simulink model "Coil5"  (Simulink 7.3)
settings: Solver=ode23tb  StartTime=0.0  StopTime=7/60  RelTol=1e-3
libraries: powerlib x163
settings Model: Creator=DIVYA  LastModifiedBy=intel

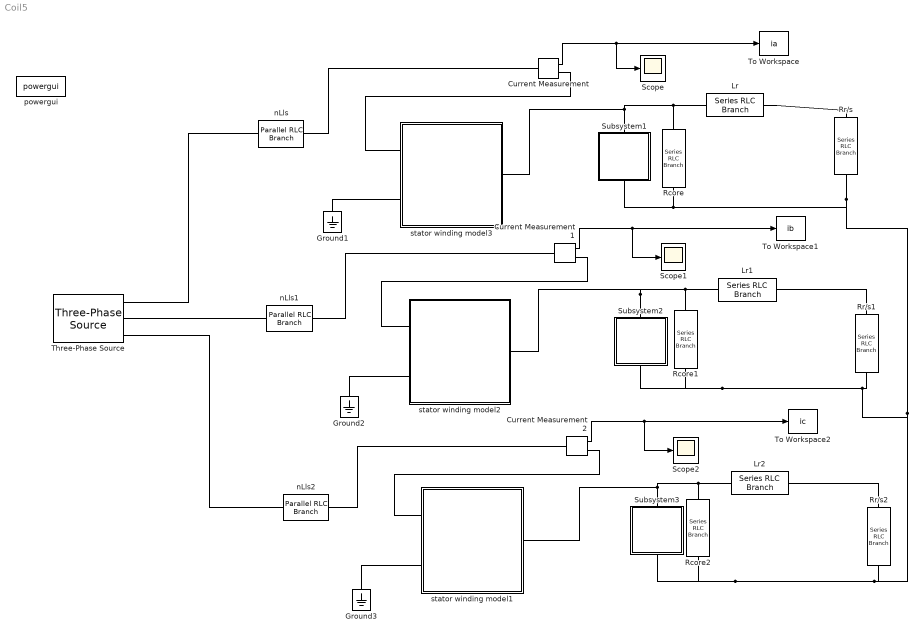
== system Coil5 ==
  Current Measurement : powerlib/Measurements/Current Measurement  DialogController=POWERSYS.PowerSysDialog  SystemSampleTime=-1  PhasorSimulation=off  OutputType=Complex  PSBequivalent=0
  Current Measurement1 : powerlib/Measurements/Current Measurement  DialogController=POWERSYS.PowerSysDialog  SystemSampleTime=-1  PhasorSimulation=off  OutputType=Complex  PSBequivalent=0
  Current Measurement2 : powerlib/Measurements/Current Measurement  DialogController=POWERSYS.PowerSysDialog  SystemSampleTime=-1  PhasorSimulation=off  OutputType=Complex  PSBequivalent=0
  Ground1 : powerlib/Elements/Ground  DialogController=POWERSYS.PowerSysDialog  PhysicalDomain=powersysdomain  SubClassName=unknown  LeftPortType=p1  RightPortType=p1  LConnTagsString=a
  Ground2 : powerlib/Elements/Ground  DialogController=POWERSYS.PowerSysDialog  PhysicalDomain=powersysdomain  SubClassName=unknown  LeftPortType=p1  RightPortType=p1  LConnTagsString=a
  Ground3 : powerlib/Elements/Ground  DialogController=POWERSYS.PowerSysDialog  PhysicalDomain=powersysdomain  SubClassName=unknown  LeftPortType=p1  RightPortType=p1  LConnTagsString=a
  Lr : powerlib/Elements/Series RLC Branch  DialogController=POWERSYS.PowerSysDialog  PhysicalDomain=powersysdomain  SubClassName=unknown  LeftPortType=p1  RightPortType=p1  LConnTagsString=__new0  RConnTagsString=__new0  BranchType=L  Resistance=1.0  Inductance=15.04e-3  SetiL0=off  InitialCurrent=0  Capacitance=1.0  Setx0=off  InitialVoltage=0  Measurements=None
  Lr1 : powerlib/Elements/Series RLC Branch  DialogController=POWERSYS.PowerSysDialog  PhysicalDomain=powersysdomain  SubClassName=unknown  LeftPortType=p1  RightPortType=p1  LConnTagsString=__new0  RConnTagsString=__new0  BranchType=L  Resistance=1.0  Inductance=15.04e-3  SetiL0=off  InitialCurrent=0  Capacitance=1.0  Setx0=off  InitialVoltage=0  Measurements=None
  Lr2 : powerlib/Elements/Series RLC Branch  DialogController=POWERSYS.PowerSysDialog  PhysicalDomain=powersysdomain  SubClassName=unknown  LeftPortType=p1  RightPortType=p1  LConnTagsString=__new0  RConnTagsString=__new0  BranchType=L  Resistance=1.0  Inductance=15.04e-3  SetiL0=off  InitialCurrent=0  Capacitance=1.0  Setx0=off  InitialVoltage=0  Measurements=None
  Rcore : powerlib/Elements/Series RLC Branch  DialogController=POWERSYS.PowerSysDialog  PhysicalDomain=powersysdomain  SubClassName=unknown  LeftPortType=p1  RightPortType=p1  LConnTagsString=__new0  RConnTagsString=__new0  BranchType=R  Resistance=2568  Inductance=1.0  SetiL0=off  InitialCurrent=0  Capacitance=1.0  Setx0=off  InitialVoltage=0  Measurements=None
  Rcore1 : powerlib/Elements/Series RLC Branch  DialogController=POWERSYS.PowerSysDialog  PhysicalDomain=powersysdomain  SubClassName=unknown  LeftPortType=p1  RightPortType=p1  LConnTagsString=__new0  RConnTagsString=__new0  BranchType=R  Resistance=2568  Inductance=1.0  SetiL0=off  InitialCurrent=0  Capacitance=1.0  Setx0=off  InitialVoltage=0  Measurements=None
  Rcore2 : powerlib/Elements/Series RLC Branch  DialogController=POWERSYS.PowerSysDialog  PhysicalDomain=powersysdomain  SubClassName=unknown  LeftPortType=p1  RightPortType=p1  LConnTagsString=__new0  RConnTagsString=__new0  BranchType=R  Resistance=2568  Inductance=1.0  SetiL0=off  InitialCurrent=0  Capacitance=1.0  Setx0=off  InitialVoltage=0  Measurements=None
  Rr/s : powerlib/Elements/Series RLC Branch  DialogController=POWERSYS.PowerSysDialog  PhysicalDomain=powersysdomain  SubClassName=unknown  LeftPortType=p1  RightPortType=p1  LConnTagsString=__new0  RConnTagsString=__new0  BranchType=R  Resistance=1.28/0.027  Inductance=1.0  SetiL0=off  InitialCurrent=0  Capacitance=1.0  Setx0=off  InitialVoltage=0  Measurements=None
  Rr/s1 : powerlib/Elements/Series RLC Branch  DialogController=POWERSYS.PowerSysDialog  PhysicalDomain=powersysdomain  SubClassName=unknown  LeftPortType=p1  RightPortType=p1  LConnTagsString=__new0  RConnTagsString=__new0  BranchType=R  Resistance=1.28/0.027  Inductance=1.0  SetiL0=off  InitialCurrent=0  Capacitance=1.0  Setx0=off  InitialVoltage=0  Measurements=None
  Rr/s2 : powerlib/Elements/Series RLC Branch  DialogController=POWERSYS.PowerSysDialog  PhysicalDomain=powersysdomain  SubClassName=unknown  LeftPortType=p1  RightPortType=p1  LConnTagsString=__new0  RConnTagsString=__new0  BranchType=R  Resistance=1.28/0.027  Inductance=1.0  SetiL0=off  InitialCurrent=0  Capacitance=1.0  Setx0=off  InitialVoltage=0  Measurements=None
  Scope : Scope
      settings: YMin=-8  YMax=6  SaveName=ScopeData18
  Scope1 : Scope
      settings: SaveName=ScopeData6
  Scope2 : Scope
      settings: SaveName=ScopeData7
  Subsystem1 : Subsystem
  Subsystem2 : Subsystem
  Subsystem3 : Subsystem
  Three-Phase Source : powerlib/Electrical Sources/Three-Phase Source  DialogController=POWERSYS.PowerSysDialog  SystemSampleTime=-1  Voltage=460  PhaseAngle=0  Frequency=60  InternalConnection=Yg  SpecifyImpedance=on  Resistance=0.8929  Inductance=16.58e-3  ShortCircuitLevel=100e6  BaseVoltage=25e3  XRratio=7
  To Workspace : ToWorkspace  VariableName=ia  SampleTime=1/(60*128)  SaveFormat=Array
  To Workspace1 : ToWorkspace  VariableName=ib  SampleTime=1/(60*128)  SaveFormat=Array
  To Workspace2 : ToWorkspace  VariableName=ic  SampleTime=1/(60*128)  SaveFormat=Array
  nLls : powerlib/Elements/Parallel RLC Branch  DialogController=POWERSYS.PowerSysDialog  PhysicalDomain=powersysdomain  SubClassName=unknown  LeftPortType=p1  RightPortType=p1  LConnTagsString=a  RConnTagsString=__new0  BranchType=L  Resistance=1.0  Inductance=4.926e-6  SetiL0=off  InitialCurrent=0  Capacitance=1.0  Setx0=off  InitialVoltage=0  Measurements=None
  nLls1 : powerlib/Elements/Parallel RLC Branch  DialogController=POWERSYS.PowerSysDialog  PhysicalDomain=powersysdomain  SubClassName=unknown  LeftPortType=p1  RightPortType=p1  LConnTagsString=a  RConnTagsString=__new0  BranchType=L  Resistance=1.0  Inductance=4.926e-6  SetiL0=off  InitialCurrent=0  Capacitance=1.0  Setx0=off  InitialVoltage=0  Measurements=None
  nLls2 : powerlib/Elements/Parallel RLC Branch  DialogController=POWERSYS.PowerSysDialog  PhysicalDomain=powersysdomain  SubClassName=unknown  LeftPortType=p1  RightPortType=p1  LConnTagsString=a  RConnTagsString=__new0  BranchType=L  Resistance=1.0  Inductance=4.926e-6  SetiL0=off  InitialCurrent=0  Capacitance=1.0  Setx0=off  InitialVoltage=0  Measurements=None
  powergui : powerlib/powergui  SystemSampleTime=-1  SimulationMode=Continuous  SampleTime=50e-6  frequency=60  SPID=off  DisableSnubberDevices=off  DisableRonSwitches=off  DisableVfSwitches=off  SwTol=0  Interpol=off  frequencyindice=60  echomessages=off  HookPort=off  DisplayEquations=off  FunctionMessages=off  EnableUseOfTLC=off  x0status=blocks  RestoreLinks=warning  Frange=[0:2:500]  Ylog=off  Xlog=on  ShowGrid=off  save=off  variable=ZData  structure=ScopeData18  ZoomFFT=off  StartTime=0.00  cycles=2  DisplayStyle=1  fundamental=60  FreqAxis=off  MaxFrequency=200  frequencyindicesteady=1  RmsSteady=1  display=off  Ts=0  methode=off
  stator winding model1 : Subsystem
  stator winding model2 : Subsystem
  stator winding model3 : Subsystem
  wires:
  Current Measurement/1 -> To Workspace/1, Scope/1
  Current Measurement1/1 -> To Workspace1/1, Scope1/1
  Current Measurement2/1 -> To Workspace2/1, Scope2/1
  connections:
  Lr/LConn1 -- Rr/s/LConn1
  Current Measurement/LConn1 -- nLls/RConn1
  Current Measurement/RConn1 -- stator winding model3/LConn1
  Three-Phase Source/RConn1 -- nLls/LConn1
  stator winding model3/RConn1 -- Subsystem1/LConn1 -- Lr/RConn1 -- Rcore/LConn1
  stator winding model2/RConn1 -- Subsystem2/LConn1 -- Rcore1/LConn1 -- Lr1/RConn1
  Lr1/LConn1 -- Rr/s1/LConn1
  Current Measurement1/LConn1 -- nLls1/RConn1
  Current Measurement1/RConn1 -- stator winding model2/LConn1
  Ground2/LConn1 -- stator winding model2/LConn2
  Rr/s/RConn1 -- Subsystem2/RConn1 -- Rcore1/RConn1 -- Rr/s1/RConn1 -- Rr/s2/RConn1 -- Rcore2/RConn1 -- Subsystem3/RConn1 -- Subsystem1/RConn1 -- Rcore/RConn1
  stator winding model1/RConn1 -- Subsystem3/LConn1 -- Rcore2/LConn1 -- Lr2/RConn1
  Lr2/LConn1 -- Rr/s2/LConn1
  Current Measurement2/LConn1 -- nLls2/RConn1
  Current Measurement2/RConn1 -- stator winding model1/LConn1
  Ground3/LConn1 -- stator winding model1/LConn2
  Three-Phase Source/RConn2 -- nLls1/LConn1
  Three-Phase Source/RConn3 -- nLls2/LConn1
  Ground1/LConn1 -- stator winding model3/LConn2

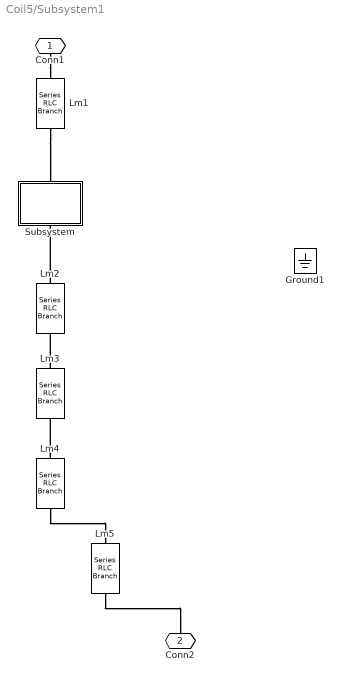
== system Coil5/Subsystem1 ==
  Ground1 : powerlib/Elements/Ground  DialogController=POWERSYS.PowerSysDialog  PhysicalDomain=powersysdomain  SubClassName=unknown  LeftPortType=p1  RightPortType=p1  LConnTagsString=a
  Lm{1..5} (5 alike) : powerlib/Elements/Series RLC Branch  DialogController=POWERSYS.PowerSysDialog  PhysicalDomain=powersysdomain  SubClassName=unknown  LeftPortType=p1  RightPortType=p1  LConnTagsString=__new0  RConnTagsString=__new0  BranchType=L  Resistance=1.0  Inductance=319e-3/6  SetiL0=off  InitialCurrent=0  Capacitance=1.0  Setx0=off  InitialVoltage=0  Measurements=None
  Subsystem : Subsystem
  Conn1 : PMIOPort  Port=1  Side=Left
  Conn2 : PMIOPort  Port=2  Side=Right
  connections:
  Conn1/RConn1 -- Lm1/LConn1
  Lm4/LConn1 -- Lm3/RConn1
  Lm3/LConn1 -- Lm2/RConn1
  Lm2/LConn1 -- Subsystem/RConn1
  Lm1/RConn1 -- Subsystem/LConn1
  Lm4/RConn1 -- Lm5/LConn1
  Lm5/RConn1 -- Conn2/RConn1

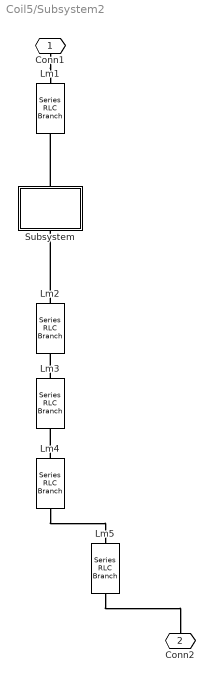
== system Coil5/Subsystem2 ==
  Lm{1..5} (5 alike) : powerlib/Elements/Series RLC Branch  DialogController=POWERSYS.PowerSysDialog  PhysicalDomain=powersysdomain  SubClassName=unknown  LeftPortType=p1  RightPortType=p1  LConnTagsString=__new0  RConnTagsString=__new0  BranchType=L  Resistance=1.0  Inductance=319e-3/6  SetiL0=off  InitialCurrent=0  Capacitance=1.0  Setx0=off  InitialVoltage=0  Measurements=None
  Subsystem : Subsystem
  Conn1 : PMIOPort  Port=1  Side=Left
  Conn2 : PMIOPort  Port=2  Side=Right
  connections:
  Conn1/RConn1 -- Lm1/LConn1
  Lm4/LConn1 -- Lm3/RConn1
  Lm3/LConn1 -- Lm2/RConn1
  Lm2/LConn1 -- Subsystem/RConn1
  Subsystem/LConn1 -- Lm1/RConn1
  Lm4/RConn1 -- Lm5/LConn1
  Lm5/RConn1 -- Conn2/RConn1

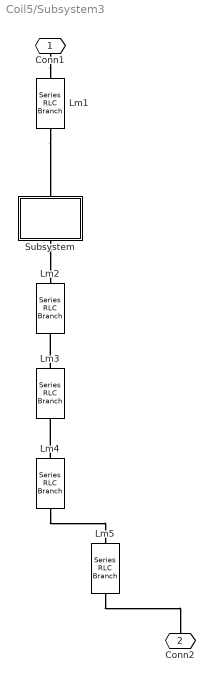
== system Coil5/Subsystem3 ==
  Lm{1..5} (5 alike) : powerlib/Elements/Series RLC Branch  DialogController=POWERSYS.PowerSysDialog  PhysicalDomain=powersysdomain  SubClassName=unknown  LeftPortType=p1  RightPortType=p1  LConnTagsString=__new0  RConnTagsString=__new0  BranchType=L  Resistance=1.0  Inductance=319e-3/6  SetiL0=off  InitialCurrent=0  Capacitance=1.0  Setx0=off  InitialVoltage=0  Measurements=None
  Subsystem : Subsystem
  Conn1 : PMIOPort  Port=1  Side=Left
  Conn2 : PMIOPort  Port=2  Side=Right
  connections:
  Conn1/RConn1 -- Lm1/LConn1
  Lm4/LConn1 -- Lm3/RConn1
  Lm3/LConn1 -- Lm2/RConn1
  Subsystem/RConn1 -- Lm2/LConn1
  Lm1/RConn1 -- Subsystem/LConn1
  Lm4/RConn1 -- Lm5/LConn1
  Lm5/RConn1 -- Conn2/RConn1

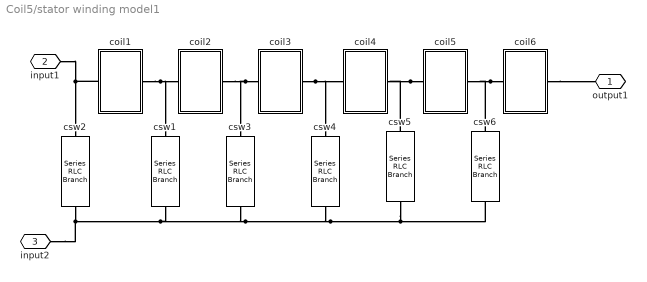
== system Coil5/stator winding model1 ==
  coil1 : Subsystem
  coil2 : Subsystem
  coil3 : Subsystem
  coil4 : Subsystem
  coil5 : Subsystem
  coil6 : Subsystem
  csw{1..6} (6 alike) : powerlib/Elements/Series RLC Branch  DialogController=POWERSYS.PowerSysDialog  PhysicalDomain=powersysdomain  SubClassName=unknown  LeftPortType=p1  RightPortType=p1  LConnTagsString=__new0  RConnTagsString=__new0  BranchType=RC  Resistance=(4*10)/(192*6)  Inductance=1.0  SetiL0=off  InitialCurrent=0  Capacitance=0.213e-9/6  Setx0=off  InitialVoltage=0  Measurements=None
  output1 : PMIOPort  Port=1  Side=Left
  input1 : PMIOPort  Port=2  Side=Right
  input2 : PMIOPort  Port=3  Side=Left
  connections:
  coil1/RConn1 -- coil2/LConn1 -- csw1/LConn1
  coil3/LConn1 -- coil2/RConn1 -- csw3/LConn1
  coil3/RConn1 -- coil4/LConn1 -- csw4/LConn1
  coil5/LConn1 -- csw5/LConn1 -- coil4/RConn1
  coil6/LConn1 -- csw6/LConn1 -- coil5/RConn1
  input2/RConn1 -- csw6/RConn1 -- csw5/RConn1 -- csw4/RConn1 -- csw3/RConn1 -- csw1/RConn1 -- csw2/RConn1
  coil6/RConn1 -- output1/RConn1
  coil1/LConn1 -- csw2/LConn1 -- input1/RConn1

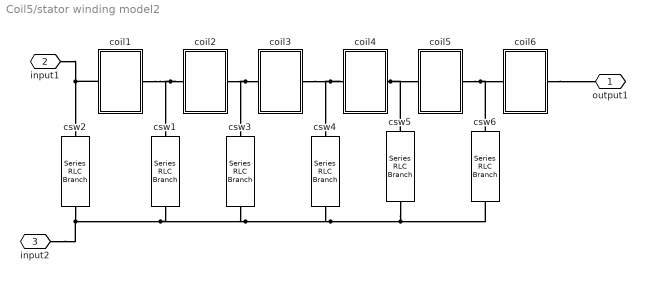
== system Coil5/stator winding model2 ==
  coil1 : Subsystem
  coil2 : Subsystem
  coil3 : Subsystem
  coil4 : Subsystem
  coil5 : Subsystem
  coil6 : Subsystem
  csw{1..6} (6 alike) : powerlib/Elements/Series RLC Branch  DialogController=POWERSYS.PowerSysDialog  PhysicalDomain=powersysdomain  SubClassName=unknown  LeftPortType=p1  RightPortType=p1  LConnTagsString=__new0  RConnTagsString=__new0  BranchType=RC  Resistance=(4*10)/(192*6)  Inductance=1.0  SetiL0=off  InitialCurrent=0  Capacitance=0.213e-9/6  Setx0=off  InitialVoltage=0  Measurements=None
  output1 : PMIOPort  Port=1  Side=Left
  input1 : PMIOPort  Port=2  Side=Right
  input2 : PMIOPort  Port=3  Side=Left
  connections:
  coil2/LConn1 -- csw1/LConn1 -- coil1/RConn1
  coil3/LConn1 -- csw3/LConn1 -- coil2/RConn1
  coil4/LConn1 -- csw4/LConn1 -- coil3/RConn1
  coil4/RConn1 -- csw5/LConn1 -- coil5/LConn1
  coil5/RConn1 -- coil6/LConn1 -- csw6/LConn1
  input2/RConn1 -- csw6/RConn1 -- csw5/RConn1 -- csw4/RConn1 -- csw3/RConn1 -- csw1/RConn1 -- csw2/RConn1
  coil6/RConn1 -- output1/RConn1
  coil1/LConn1 -- csw2/LConn1 -- input1/RConn1

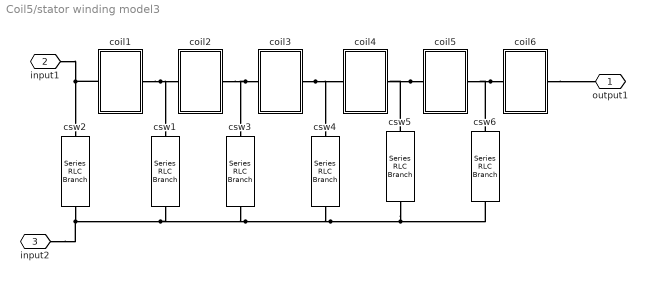
== system Coil5/stator winding model3 ==
  coil1 : Subsystem
  coil2 : Subsystem
  coil3 : Subsystem
  coil4 : Subsystem
  coil5 : Subsystem
  coil6 : Subsystem
  csw{1..6} (6 alike) : powerlib/Elements/Series RLC Branch  DialogController=POWERSYS.PowerSysDialog  PhysicalDomain=powersysdomain  SubClassName=unknown  LeftPortType=p1  RightPortType=p1  LConnTagsString=__new0  RConnTagsString=__new0  BranchType=RC  Resistance=(4*10)/(192*6)  Inductance=1.0  SetiL0=off  InitialCurrent=0  Capacitance=0.213e-9/6  Setx0=off  InitialVoltage=0  Measurements=None
  output1 : PMIOPort  Port=1  Side=Left
  input1 : PMIOPort  Port=2  Side=Right
  input2 : PMIOPort  Port=3  Side=Left
  connections:
  coil1/RConn1 -- coil2/LConn1 -- csw1/LConn1
  coil3/LConn1 -- coil2/RConn1 -- csw3/LConn1
  coil3/RConn1 -- coil4/LConn1 -- csw4/LConn1
  coil5/LConn1 -- csw5/LConn1 -- coil4/RConn1
  coil6/LConn1 -- csw6/LConn1 -- coil5/RConn1
  input2/RConn1 -- csw6/RConn1 -- csw5/RConn1 -- csw4/RConn1 -- csw3/RConn1 -- csw1/RConn1 -- csw2/RConn1
  coil6/RConn1 -- output1/RConn1
  coil1/LConn1 -- csw2/LConn1 -- input1/RConn1

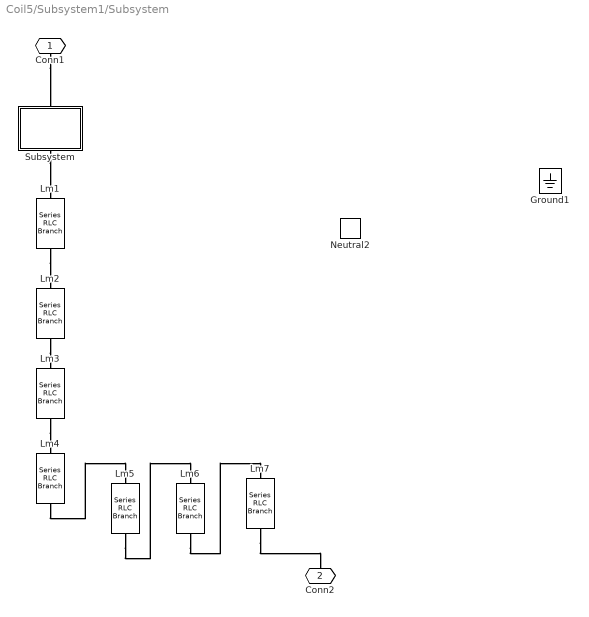
== system Coil5/Subsystem1/Subsystem ==
  Ground1 : powerlib/Elements/Ground  DialogController=POWERSYS.PowerSysDialog  PhysicalDomain=powersysdomain  SubClassName=unknown  LeftPortType=p1  RightPortType=p1  LConnTagsString=a
  Lm{1..7} (7 alike) : powerlib/Elements/Series RLC Branch  DialogController=POWERSYS.PowerSysDialog  PhysicalDomain=powersysdomain  SubClassName=unknown  LeftPortType=p1  RightPortType=p1  LConnTagsString=__new0  RConnTagsString=__new0  BranchType=L  Resistance=1.0  Inductance=319e-3/(8*6)  SetiL0=off  InitialCurrent=0  Capacitance=1.0  Setx0=off  InitialVoltage=0  Measurements=None
  Neutral2 : powerlib/Elements/Neutral  DialogController=POWERSYS.PowerSysDialog  PhysicalDomain=powersysdomain  SubClassName=unknown  LeftPortType=p1  RightPortType=p1  LConnTagsString=a  NodeNumber=20
  Subsystem : Subsystem
  Conn1 : PMIOPort  Port=1  Side=Left
  Conn2 : PMIOPort  Port=2  Side=Right
  connections:
  Lm1/RConn1 -- Lm2/LConn1
  Lm2/RConn1 -- Lm3/LConn1
  Lm3/RConn1 -- Lm4/LConn1
  Lm4/RConn1 -- Lm5/RConn1
  Lm5/LConn1 -- Lm6/RConn1
  Lm6/LConn1 -- Lm7/LConn1
  Lm7/RConn1 -- Conn2/RConn1
  Conn1/RConn1 -- Subsystem/LConn1
  Subsystem/RConn1 -- Lm1/LConn1

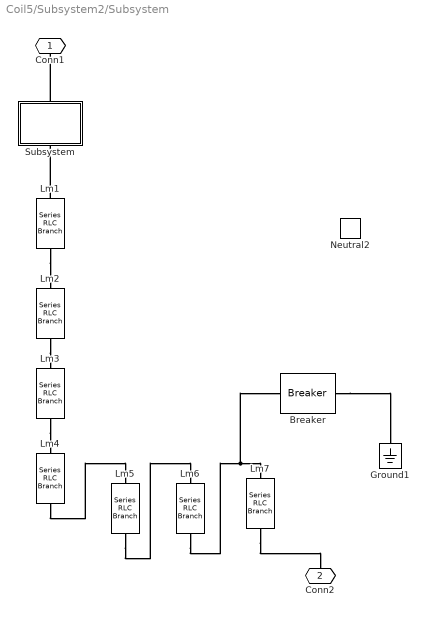
== system Coil5/Subsystem2/Subsystem ==
  Breaker : powerlib/Elements/Breaker  DialogController=POWERSYS.PowerSysDialog  SystemSampleTime=-1  BreakerResistance=0.01  InitialState=0  SnubberResistance=1e6  SnubberCapacitance=inf  SwitchingTimes="[ 3/60  20/60 ]"  External=off  Measurements=None  MoreParameters=off  NoBreakLoop=off
  Ground1 : powerlib/Elements/Ground  DialogController=POWERSYS.PowerSysDialog  PhysicalDomain=powersysdomain  SubClassName=unknown  LeftPortType=p1  RightPortType=p1  LConnTagsString=a
  Lm{1..7} (7 alike) : powerlib/Elements/Series RLC Branch  DialogController=POWERSYS.PowerSysDialog  PhysicalDomain=powersysdomain  SubClassName=unknown  LeftPortType=p1  RightPortType=p1  LConnTagsString=__new0  RConnTagsString=__new0  BranchType=L  Resistance=1.0  Inductance=319e-3/(8*6)  SetiL0=off  InitialCurrent=0  Capacitance=1.0  Setx0=off  InitialVoltage=0  Measurements=None
  Neutral2 : powerlib/Elements/Neutral  DialogController=POWERSYS.PowerSysDialog  PhysicalDomain=powersysdomain  SubClassName=unknown  LeftPortType=p1  RightPortType=p1  LConnTagsString=a  NodeNumber=20
  Subsystem : Subsystem
  Conn1 : PMIOPort  Port=1  Side=Left
  Conn2 : PMIOPort  Port=2  Side=Right
  connections:
  Lm1/RConn1 -- Lm2/LConn1
  Lm2/RConn1 -- Lm3/LConn1
  Lm3/RConn1 -- Lm4/LConn1
  Lm4/RConn1 -- Lm5/RConn1
  Lm5/LConn1 -- Lm6/RConn1
  Lm6/LConn1 -- Lm7/LConn1 -- Breaker/LConn1
  Lm7/RConn1 -- Conn2/RConn1
  Subsystem/LConn1 -- Conn1/RConn1
  Lm1/LConn1 -- Subsystem/RConn1
  Breaker/RConn1 -- Ground1/LConn1

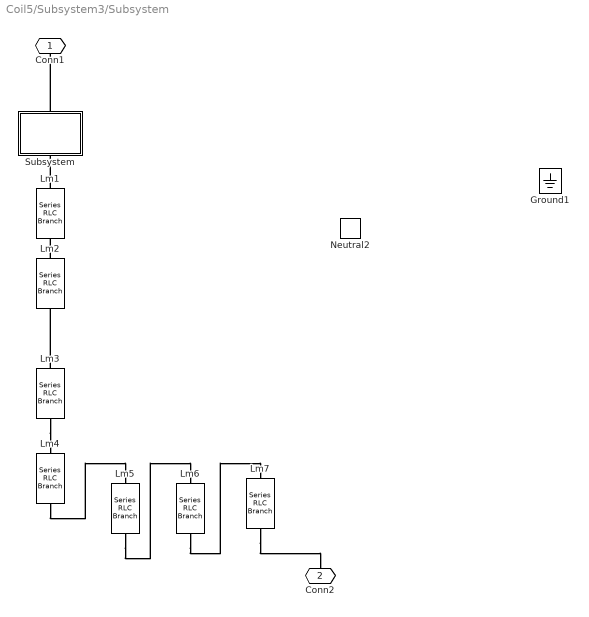
== system Coil5/Subsystem3/Subsystem ==
  Ground1 : powerlib/Elements/Ground  DialogController=POWERSYS.PowerSysDialog  PhysicalDomain=powersysdomain  SubClassName=unknown  LeftPortType=p1  RightPortType=p1  LConnTagsString=a
  Lm{1..7} (7 alike) : powerlib/Elements/Series RLC Branch  DialogController=POWERSYS.PowerSysDialog  PhysicalDomain=powersysdomain  SubClassName=unknown  LeftPortType=p1  RightPortType=p1  LConnTagsString=__new0  RConnTagsString=__new0  BranchType=L  Resistance=1.0  Inductance=319e-3/(8*6)  SetiL0=off  InitialCurrent=0  Capacitance=1.0  Setx0=off  InitialVoltage=0  Measurements=None
  Neutral2 : powerlib/Elements/Neutral  DialogController=POWERSYS.PowerSysDialog  PhysicalDomain=powersysdomain  SubClassName=unknown  LeftPortType=p1  RightPortType=p1  LConnTagsString=a  NodeNumber=20
  Subsystem : Subsystem
  Conn1 : PMIOPort  Port=1  Side=Left
  Conn2 : PMIOPort  Port=2  Side=Right
  connections:
  Lm2/LConn1 -- Lm1/RConn1
  Lm3/LConn1 -- Lm2/RConn1
  Lm3/RConn1 -- Lm4/LConn1
  Lm4/RConn1 -- Lm5/RConn1
  Lm5/LConn1 -- Lm6/RConn1
  Lm6/LConn1 -- Lm7/LConn1
  Lm7/RConn1 -- Conn2/RConn1
  Subsystem/LConn1 -- Conn1/RConn1
  Lm1/LConn1 -- Subsystem/RConn1

== system Coil5/stator winding model1/coil1 ==
  Ground : powerlib/Elements/Ground  DialogController=POWERSYS.PowerSysDialog  PhysicalDomain=powersysdomain  SubClassName=unknown  LeftPortType=p1  RightPortType=p1  LConnTagsString=a
  LC Branch1 : powerlib/Elements/Parallel RLC Branch  DialogController=POWERSYS.PowerSysDialog  PhysicalDomain=powersysdomain  SubClassName=unknown  LeftPortType=p1  RightPortType=p1  LConnTagsString=a  RConnTagsString=__new0  BranchType=RLC  Resistance=11.867e3/6  Inductance=(11.35E-3)/6  SetiL0=off  InitialCurrent=0  Capacitance=0.852e-9*6  Setx0=off  InitialVoltage=0  Measurements=None
  Rs1 : powerlib/Elements/Parallel RLC Branch  DialogController=POWERSYS.PowerSysDialog  PhysicalDomain=powersysdomain  SubClassName=unknown  LeftPortType=p1  RightPortType=p1  LConnTagsString=a  RConnTagsString=__new0  BranchType=R  Resistance=1.41/6  Inductance=1.0  SetiL0=off  InitialCurrent=0  Capacitance=1.0  Setx0=off  InitialVoltage=0  Measurements=None
  Conn1 : PMIOPort  Port=1  Side=Left
  Conn2 : PMIOPort  Port=2  Side=Right
  connections:
  Rs1/LConn1 -- Conn1/RConn1
  LC Branch1/RConn1 -- Conn2/RConn1
  Rs1/RConn1 -- LC Branch1/LConn1

== system Coil5/stator winding model1/coil2 ==
  Ground : powerlib/Elements/Ground  DialogController=POWERSYS.PowerSysDialog  PhysicalDomain=powersysdomain  SubClassName=unknown  LeftPortType=p1  RightPortType=p1  LConnTagsString=a
  LC Branch1 : powerlib/Elements/Parallel RLC Branch  DialogController=POWERSYS.PowerSysDialog  PhysicalDomain=powersysdomain  SubClassName=unknown  LeftPortType=p1  RightPortType=p1  LConnTagsString=a  RConnTagsString=__new0  BranchType=RLC  Resistance=11.867e3/6  Inductance=(11.35E-3)/6  SetiL0=off  InitialCurrent=0  Capacitance=0.852e-9*6  Setx0=off  InitialVoltage=0  Measurements=None
  Rs1 : powerlib/Elements/Parallel RLC Branch  DialogController=POWERSYS.PowerSysDialog  PhysicalDomain=powersysdomain  SubClassName=unknown  LeftPortType=p1  RightPortType=p1  LConnTagsString=a  RConnTagsString=__new0  BranchType=R  Resistance=1.41/6  Inductance=1.0  SetiL0=off  InitialCurrent=0  Capacitance=1.0  Setx0=off  InitialVoltage=0  Measurements=None
  Conn1 : PMIOPort  Port=1  Side=Left
  Conn2 : PMIOPort  Port=2  Side=Right
  connections:
  Rs1/LConn1 -- Conn1/RConn1
  LC Branch1/RConn1 -- Conn2/RConn1
  Rs1/RConn1 -- LC Branch1/LConn1

== system Coil5/stator winding model1/coil3 ==
  Ground : powerlib/Elements/Ground  DialogController=POWERSYS.PowerSysDialog  PhysicalDomain=powersysdomain  SubClassName=unknown  LeftPortType=p1  RightPortType=p1  LConnTagsString=a
  LC Branch1 : powerlib/Elements/Parallel RLC Branch  DialogController=POWERSYS.PowerSysDialog  PhysicalDomain=powersysdomain  SubClassName=unknown  LeftPortType=p1  RightPortType=p1  LConnTagsString=a  RConnTagsString=__new0  BranchType=RLC  Resistance=11.867e3/6  Inductance=(11.35E-3)/6  SetiL0=off  InitialCurrent=0  Capacitance=0.852e-9*6  Setx0=off  InitialVoltage=0  Measurements=None
  Rs1 : powerlib/Elements/Parallel RLC Branch  DialogController=POWERSYS.PowerSysDialog  PhysicalDomain=powersysdomain  SubClassName=unknown  LeftPortType=p1  RightPortType=p1  LConnTagsString=a  RConnTagsString=__new0  BranchType=R  Resistance=1.41/6  Inductance=1.0  SetiL0=off  InitialCurrent=0  Capacitance=1.0  Setx0=off  InitialVoltage=0  Measurements=None
  Conn1 : PMIOPort  Port=1  Side=Left
  Conn2 : PMIOPort  Port=2  Side=Right
  connections:
  Rs1/LConn1 -- Conn1/RConn1
  LC Branch1/RConn1 -- Conn2/RConn1
  Rs1/RConn1 -- LC Branch1/LConn1

== system Coil5/stator winding model1/coil4 ==
  Ground : powerlib/Elements/Ground  DialogController=POWERSYS.PowerSysDialog  PhysicalDomain=powersysdomain  SubClassName=unknown  LeftPortType=p1  RightPortType=p1  LConnTagsString=a
  LC Branch1 : powerlib/Elements/Parallel RLC Branch  DialogController=POWERSYS.PowerSysDialog  PhysicalDomain=powersysdomain  SubClassName=unknown  LeftPortType=p1  RightPortType=p1  LConnTagsString=a  RConnTagsString=__new0  BranchType=RLC  Resistance=11.867e3/6  Inductance=(11.35E-3)/6  SetiL0=off  InitialCurrent=0  Capacitance=0.852e-9*6  Setx0=off  InitialVoltage=0  Measurements=None
  Rs1 : powerlib/Elements/Parallel RLC Branch  DialogController=POWERSYS.PowerSysDialog  PhysicalDomain=powersysdomain  SubClassName=unknown  LeftPortType=p1  RightPortType=p1  LConnTagsString=a  RConnTagsString=__new0  BranchType=R  Resistance=1.41/6  Inductance=1.0  SetiL0=off  InitialCurrent=0  Capacitance=1.0  Setx0=off  InitialVoltage=0  Measurements=None
  Conn1 : PMIOPort  Port=1  Side=Left
  Conn2 : PMIOPort  Port=2  Side=Right
  connections:
  Rs1/LConn1 -- Conn1/RConn1
  LC Branch1/RConn1 -- Conn2/RConn1
  Rs1/RConn1 -- LC Branch1/LConn1

== system Coil5/stator winding model1/coil5 ==
  Ground : powerlib/Elements/Ground  DialogController=POWERSYS.PowerSysDialog  PhysicalDomain=powersysdomain  SubClassName=unknown  LeftPortType=p1  RightPortType=p1  LConnTagsString=a
  LC Branch1 : powerlib/Elements/Parallel RLC Branch  DialogController=POWERSYS.PowerSysDialog  PhysicalDomain=powersysdomain  SubClassName=unknown  LeftPortType=p1  RightPortType=p1  LConnTagsString=a  RConnTagsString=__new0  BranchType=RLC  Resistance=11.867e3/6  Inductance=(11.35E-3)/6  SetiL0=off  InitialCurrent=0  Capacitance=0.852e-9*6  Setx0=off  InitialVoltage=0  Measurements=None
  Rs1 : powerlib/Elements/Parallel RLC Branch  DialogController=POWERSYS.PowerSysDialog  PhysicalDomain=powersysdomain  SubClassName=unknown  LeftPortType=p1  RightPortType=p1  LConnTagsString=a  RConnTagsString=__new0  BranchType=R  Resistance=1.41/6  Inductance=1.0  SetiL0=off  InitialCurrent=0  Capacitance=1.0  Setx0=off  InitialVoltage=0  Measurements=None
  Conn1 : PMIOPort  Port=1  Side=Left
  Conn2 : PMIOPort  Port=2  Side=Right
  connections:
  Rs1/LConn1 -- Conn1/RConn1
  LC Branch1/RConn1 -- Conn2/RConn1
  Rs1/RConn1 -- LC Branch1/LConn1

== system Coil5/stator winding model1/coil6 ==
  Ground : powerlib/Elements/Ground  DialogController=POWERSYS.PowerSysDialog  PhysicalDomain=powersysdomain  SubClassName=unknown  LeftPortType=p1  RightPortType=p1  LConnTagsString=a
  LC Branch1 : powerlib/Elements/Parallel RLC Branch  DialogController=POWERSYS.PowerSysDialog  PhysicalDomain=powersysdomain  SubClassName=unknown  LeftPortType=p1  RightPortType=p1  LConnTagsString=a  RConnTagsString=__new0  BranchType=RLC  Resistance=11.867e3/6  Inductance=(11.35E-3)/6  SetiL0=off  InitialCurrent=0  Capacitance=0.852e-9*6  Setx0=off  InitialVoltage=0  Measurements=None
  Rs1 : powerlib/Elements/Parallel RLC Branch  DialogController=POWERSYS.PowerSysDialog  PhysicalDomain=powersysdomain  SubClassName=unknown  LeftPortType=p1  RightPortType=p1  LConnTagsString=a  RConnTagsString=__new0  BranchType=R  Resistance=1.41/6  Inductance=1.0  SetiL0=off  InitialCurrent=0  Capacitance=1.0  Setx0=off  InitialVoltage=0  Measurements=None
  Conn1 : PMIOPort  Port=1  Side=Left
  Conn2 : PMIOPort  Port=2  Side=Right
  connections:
  Rs1/LConn1 -- Conn1/RConn1
  LC Branch1/RConn1 -- Conn2/RConn1
  Rs1/RConn1 -- LC Branch1/LConn1

== system Coil5/stator winding model2/coil1 ==
  Ground : powerlib/Elements/Ground  DialogController=POWERSYS.PowerSysDialog  PhysicalDomain=powersysdomain  SubClassName=unknown  LeftPortType=p1  RightPortType=p1  LConnTagsString=a
  LC Branch1 : powerlib/Elements/Parallel RLC Branch  DialogController=POWERSYS.PowerSysDialog  PhysicalDomain=powersysdomain  SubClassName=unknown  LeftPortType=p1  RightPortType=p1  LConnTagsString=a  RConnTagsString=__new0  BranchType=RLC  Resistance=11.867e3/6  Inductance=(11.35E-3)/6  SetiL0=off  InitialCurrent=0  Capacitance=0.852e-9*6  Setx0=off  InitialVoltage=0  Measurements=None
  Rs1 : powerlib/Elements/Parallel RLC Branch  DialogController=POWERSYS.PowerSysDialog  PhysicalDomain=powersysdomain  SubClassName=unknown  LeftPortType=p1  RightPortType=p1  LConnTagsString=a  RConnTagsString=__new0  BranchType=R  Resistance=1.41/6  Inductance=1.0  SetiL0=off  InitialCurrent=0  Capacitance=1.0  Setx0=off  InitialVoltage=0  Measurements=None
  Conn1 : PMIOPort  Port=1  Side=Left
  Conn2 : PMIOPort  Port=2  Side=Right
  connections:
  Rs1/LConn1 -- Conn1/RConn1
  LC Branch1/RConn1 -- Conn2/RConn1
  Rs1/RConn1 -- LC Branch1/LConn1

== system Coil5/stator winding model2/coil2 ==
  Ground : powerlib/Elements/Ground  DialogController=POWERSYS.PowerSysDialog  PhysicalDomain=powersysdomain  SubClassName=unknown  LeftPortType=p1  RightPortType=p1  LConnTagsString=a
  LC Branch1 : powerlib/Elements/Parallel RLC Branch  DialogController=POWERSYS.PowerSysDialog  PhysicalDomain=powersysdomain  SubClassName=unknown  LeftPortType=p1  RightPortType=p1  LConnTagsString=a  RConnTagsString=__new0  BranchType=RLC  Resistance=11.867e3/6  Inductance=(11.35E-3)/6  SetiL0=off  InitialCurrent=0  Capacitance=0.852e-9*6  Setx0=off  InitialVoltage=0  Measurements=None
  Rs1 : powerlib/Elements/Parallel RLC Branch  DialogController=POWERSYS.PowerSysDialog  PhysicalDomain=powersysdomain  SubClassName=unknown  LeftPortType=p1  RightPortType=p1  LConnTagsString=a  RConnTagsString=__new0  BranchType=R  Resistance=1.41/6  Inductance=1.0  SetiL0=off  InitialCurrent=0  Capacitance=1.0  Setx0=off  InitialVoltage=0  Measurements=None
  Conn1 : PMIOPort  Port=1  Side=Left
  Conn2 : PMIOPort  Port=2  Side=Right
  connections:
  Rs1/LConn1 -- Conn1/RConn1
  LC Branch1/RConn1 -- Conn2/RConn1
  Rs1/RConn1 -- LC Branch1/LConn1

== system Coil5/stator winding model2/coil3 ==
  Ground : powerlib/Elements/Ground  DialogController=POWERSYS.PowerSysDialog  PhysicalDomain=powersysdomain  SubClassName=unknown  LeftPortType=p1  RightPortType=p1  LConnTagsString=a
  LC Branch1 : powerlib/Elements/Parallel RLC Branch  DialogController=POWERSYS.PowerSysDialog  PhysicalDomain=powersysdomain  SubClassName=unknown  LeftPortType=p1  RightPortType=p1  LConnTagsString=a  RConnTagsString=__new0  BranchType=RLC  Resistance=11.867e3/6  Inductance=(11.35E-3)/6  SetiL0=off  InitialCurrent=0  Capacitance=0.852e-9*6  Setx0=off  InitialVoltage=0  Measurements=None
  Rs1 : powerlib/Elements/Parallel RLC Branch  DialogController=POWERSYS.PowerSysDialog  PhysicalDomain=powersysdomain  SubClassName=unknown  LeftPortType=p1  RightPortType=p1  LConnTagsString=a  RConnTagsString=__new0  BranchType=R  Resistance=1.41/6  Inductance=1.0  SetiL0=off  InitialCurrent=0  Capacitance=1.0  Setx0=off  InitialVoltage=0  Measurements=None
  Conn1 : PMIOPort  Port=1  Side=Left
  Conn2 : PMIOPort  Port=2  Side=Right
  connections:
  Rs1/LConn1 -- Conn1/RConn1
  LC Branch1/RConn1 -- Conn2/RConn1
  Rs1/RConn1 -- LC Branch1/LConn1

== system Coil5/stator winding model2/coil4 ==
  Ground : powerlib/Elements/Ground  DialogController=POWERSYS.PowerSysDialog  PhysicalDomain=powersysdomain  SubClassName=unknown  LeftPortType=p1  RightPortType=p1  LConnTagsString=a
  LC Branch1 : powerlib/Elements/Parallel RLC Branch  DialogController=POWERSYS.PowerSysDialog  PhysicalDomain=powersysdomain  SubClassName=unknown  LeftPortType=p1  RightPortType=p1  LConnTagsString=a  RConnTagsString=__new0  BranchType=RLC  Resistance=11.867e3/6  Inductance=(11.35E-3)/6  SetiL0=off  InitialCurrent=0  Capacitance=0.852e-9*6  Setx0=off  InitialVoltage=0  Measurements=None
  Rs1 : powerlib/Elements/Parallel RLC Branch  DialogController=POWERSYS.PowerSysDialog  PhysicalDomain=powersysdomain  SubClassName=unknown  LeftPortType=p1  RightPortType=p1  LConnTagsString=a  RConnTagsString=__new0  BranchType=R  Resistance=1.41/6  Inductance=1.0  SetiL0=off  InitialCurrent=0  Capacitance=1.0  Setx0=off  InitialVoltage=0  Measurements=None
  Conn1 : PMIOPort  Port=1  Side=Left
  Conn2 : PMIOPort  Port=2  Side=Right
  connections:
  Rs1/LConn1 -- Conn1/RConn1
  LC Branch1/RConn1 -- Conn2/RConn1
  Rs1/RConn1 -- LC Branch1/LConn1

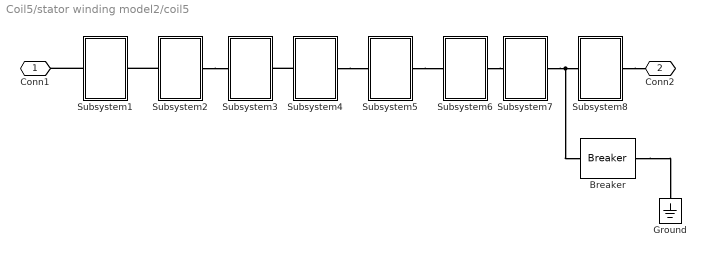
== system Coil5/stator winding model2/coil5 ==
  Breaker : powerlib/Elements/Breaker  DialogController=POWERSYS.PowerSysDialog  SystemSampleTime=-1  BreakerResistance=0.01  InitialState=0  SnubberResistance=1e6  SnubberCapacitance=inf  SwitchingTimes="[ 3/60  20/60 ]"  External=off  Measurements=None  MoreParameters=off  NoBreakLoop=off
  Ground : powerlib/Elements/Ground  DialogController=POWERSYS.PowerSysDialog  PhysicalDomain=powersysdomain  SubClassName=unknown  LeftPortType=p1  RightPortType=p1  LConnTagsString=a
  Subsystem1 : Subsystem
  Subsystem2 : Subsystem
  Subsystem3 : Subsystem
  Subsystem4 : Subsystem
  Subsystem5 : Subsystem
  Subsystem6 : Subsystem
  Subsystem7 : Subsystem
  Subsystem8 : Subsystem
  Conn1 : PMIOPort  Port=1  Side=Left
  Conn2 : PMIOPort  Port=2  Side=Right
  connections:
  Subsystem1/LConn1 -- Conn1/RConn1
  Subsystem2/LConn1 -- Subsystem1/RConn1
  Subsystem2/RConn1 -- Subsystem3/LConn1
  Subsystem4/LConn1 -- Subsystem3/RConn1
  Subsystem4/RConn1 -- Subsystem5/LConn1
  Subsystem5/RConn1 -- Subsystem6/LConn1
  Subsystem6/RConn1 -- Subsystem7/LConn1
  Subsystem7/RConn1 -- Breaker/LConn1 -- Subsystem8/LConn1
  Subsystem8/RConn1 -- Conn2/RConn1
  Breaker/RConn1 -- Ground/LConn1

== system Coil5/stator winding model2/coil6 ==
  Ground : powerlib/Elements/Ground  DialogController=POWERSYS.PowerSysDialog  PhysicalDomain=powersysdomain  SubClassName=unknown  LeftPortType=p1  RightPortType=p1  LConnTagsString=a
  LC Branch1 : powerlib/Elements/Parallel RLC Branch  DialogController=POWERSYS.PowerSysDialog  PhysicalDomain=powersysdomain  SubClassName=unknown  LeftPortType=p1  RightPortType=p1  LConnTagsString=a  RConnTagsString=__new0  BranchType=RLC  Resistance=11.867e3/6  Inductance=(11.35E-3)/6  SetiL0=off  InitialCurrent=0  Capacitance=0.852e-9*6  Setx0=off  InitialVoltage=0  Measurements=None
  Rs1 : powerlib/Elements/Parallel RLC Branch  DialogController=POWERSYS.PowerSysDialog  PhysicalDomain=powersysdomain  SubClassName=unknown  LeftPortType=p1  RightPortType=p1  LConnTagsString=a  RConnTagsString=__new0  BranchType=R  Resistance=1.41/6  Inductance=1.0  SetiL0=off  InitialCurrent=0  Capacitance=1.0  Setx0=off  InitialVoltage=0  Measurements=None
  Conn1 : PMIOPort  Port=1  Side=Left
  Conn2 : PMIOPort  Port=2  Side=Right
  connections:
  Rs1/LConn1 -- Conn1/RConn1
  LC Branch1/RConn1 -- Conn2/RConn1
  Rs1/RConn1 -- LC Branch1/LConn1

== system Coil5/stator winding model3/coil1 ==
  Ground : powerlib/Elements/Ground  DialogController=POWERSYS.PowerSysDialog  PhysicalDomain=powersysdomain  SubClassName=unknown  LeftPortType=p1  RightPortType=p1  LConnTagsString=a
  LC Branch1 : powerlib/Elements/Parallel RLC Branch  DialogController=POWERSYS.PowerSysDialog  PhysicalDomain=powersysdomain  SubClassName=unknown  LeftPortType=p1  RightPortType=p1  LConnTagsString=a  RConnTagsString=__new0  BranchType=RLC  Resistance=11.867e3/6  Inductance=(11.35E-3)/6  SetiL0=off  InitialCurrent=0  Capacitance=0.852e-9*6  Setx0=off  InitialVoltage=0  Measurements=None
  Rs1 : powerlib/Elements/Parallel RLC Branch  DialogController=POWERSYS.PowerSysDialog  PhysicalDomain=powersysdomain  SubClassName=unknown  LeftPortType=p1  RightPortType=p1  LConnTagsString=a  RConnTagsString=__new0  BranchType=R  Resistance=1.41/6  Inductance=1.0  SetiL0=off  InitialCurrent=0  Capacitance=1.0  Setx0=off  InitialVoltage=0  Measurements=None
  Conn1 : PMIOPort  Port=1  Side=Left
  Conn2 : PMIOPort  Port=2  Side=Right
  connections:
  Rs1/LConn1 -- Conn1/RConn1
  LC Branch1/RConn1 -- Conn2/RConn1
  Rs1/RConn1 -- LC Branch1/LConn1

== system Coil5/stator winding model3/coil2 ==
  Ground : powerlib/Elements/Ground  DialogController=POWERSYS.PowerSysDialog  PhysicalDomain=powersysdomain  SubClassName=unknown  LeftPortType=p1  RightPortType=p1  LConnTagsString=a
  LC Branch1 : powerlib/Elements/Parallel RLC Branch  DialogController=POWERSYS.PowerSysDialog  PhysicalDomain=powersysdomain  SubClassName=unknown  LeftPortType=p1  RightPortType=p1  LConnTagsString=a  RConnTagsString=__new0  BranchType=RLC  Resistance=11.867e3/6  Inductance=(11.35E-3)/6  SetiL0=off  InitialCurrent=0  Capacitance=0.852e-9*6  Setx0=off  InitialVoltage=0  Measurements=None
  Rs1 : powerlib/Elements/Parallel RLC Branch  DialogController=POWERSYS.PowerSysDialog  PhysicalDomain=powersysdomain  SubClassName=unknown  LeftPortType=p1  RightPortType=p1  LConnTagsString=a  RConnTagsString=__new0  BranchType=R  Resistance=1.41/6  Inductance=1.0  SetiL0=off  InitialCurrent=0  Capacitance=1.0  Setx0=off  InitialVoltage=0  Measurements=None
  Conn1 : PMIOPort  Port=1  Side=Left
  Conn2 : PMIOPort  Port=2  Side=Right
  connections:
  Rs1/LConn1 -- Conn1/RConn1
  LC Branch1/RConn1 -- Conn2/RConn1
  Rs1/RConn1 -- LC Branch1/LConn1

== system Coil5/stator winding model3/coil3 ==
  Ground : powerlib/Elements/Ground  DialogController=POWERSYS.PowerSysDialog  PhysicalDomain=powersysdomain  SubClassName=unknown  LeftPortType=p1  RightPortType=p1  LConnTagsString=a
  LC Branch1 : powerlib/Elements/Parallel RLC Branch  DialogController=POWERSYS.PowerSysDialog  PhysicalDomain=powersysdomain  SubClassName=unknown  LeftPortType=p1  RightPortType=p1  LConnTagsString=a  RConnTagsString=__new0  BranchType=RLC  Resistance=11.867e3/6  Inductance=(11.35E-3)/6  SetiL0=off  InitialCurrent=0  Capacitance=0.852e-9*6  Setx0=off  InitialVoltage=0  Measurements=None
  Rs1 : powerlib/Elements/Parallel RLC Branch  DialogController=POWERSYS.PowerSysDialog  PhysicalDomain=powersysdomain  SubClassName=unknown  LeftPortType=p1  RightPortType=p1  LConnTagsString=a  RConnTagsString=__new0  BranchType=R  Resistance=1.41/6  Inductance=1.0  SetiL0=off  InitialCurrent=0  Capacitance=1.0  Setx0=off  InitialVoltage=0  Measurements=None
  Conn1 : PMIOPort  Port=1  Side=Left
  Conn2 : PMIOPort  Port=2  Side=Right
  connections:
  Rs1/LConn1 -- Conn1/RConn1
  LC Branch1/RConn1 -- Conn2/RConn1
  Rs1/RConn1 -- LC Branch1/LConn1

== system Coil5/stator winding model3/coil4 ==
  Ground : powerlib/Elements/Ground  DialogController=POWERSYS.PowerSysDialog  PhysicalDomain=powersysdomain  SubClassName=unknown  LeftPortType=p1  RightPortType=p1  LConnTagsString=a
  LC Branch1 : powerlib/Elements/Parallel RLC Branch  DialogController=POWERSYS.PowerSysDialog  PhysicalDomain=powersysdomain  SubClassName=unknown  LeftPortType=p1  RightPortType=p1  LConnTagsString=a  RConnTagsString=__new0  BranchType=RLC  Resistance=11.867e3/6  Inductance=(11.35E-3)/6  SetiL0=off  InitialCurrent=0  Capacitance=0.852e-9*6  Setx0=off  InitialVoltage=0  Measurements=None
  Rs1 : powerlib/Elements/Parallel RLC Branch  DialogController=POWERSYS.PowerSysDialog  PhysicalDomain=powersysdomain  SubClassName=unknown  LeftPortType=p1  RightPortType=p1  LConnTagsString=a  RConnTagsString=__new0  BranchType=R  Resistance=1.41/6  Inductance=1.0  SetiL0=off  InitialCurrent=0  Capacitance=1.0  Setx0=off  InitialVoltage=0  Measurements=None
  Conn1 : PMIOPort  Port=1  Side=Left
  Conn2 : PMIOPort  Port=2  Side=Right
  connections:
  Rs1/LConn1 -- Conn1/RConn1
  LC Branch1/RConn1 -- Conn2/RConn1
  Rs1/RConn1 -- LC Branch1/LConn1

== system Coil5/stator winding model3/coil5 ==
  Ground : powerlib/Elements/Ground  DialogController=POWERSYS.PowerSysDialog  PhysicalDomain=powersysdomain  SubClassName=unknown  LeftPortType=p1  RightPortType=p1  LConnTagsString=a
  LC Branch1 : powerlib/Elements/Parallel RLC Branch  DialogController=POWERSYS.PowerSysDialog  PhysicalDomain=powersysdomain  SubClassName=unknown  LeftPortType=p1  RightPortType=p1  LConnTagsString=a  RConnTagsString=__new0  BranchType=RLC  Resistance=11.867e3/6  Inductance=(11.35E-3)/6  SetiL0=off  InitialCurrent=0  Capacitance=0.852e-9*6  Setx0=off  InitialVoltage=0  Measurements=None
  Rs1 : powerlib/Elements/Parallel RLC Branch  DialogController=POWERSYS.PowerSysDialog  PhysicalDomain=powersysdomain  SubClassName=unknown  LeftPortType=p1  RightPortType=p1  LConnTagsString=a  RConnTagsString=__new0  BranchType=R  Resistance=1.41/6  Inductance=1.0  SetiL0=off  InitialCurrent=0  Capacitance=1.0  Setx0=off  InitialVoltage=0  Measurements=None
  Conn1 : PMIOPort  Port=1  Side=Left
  Conn2 : PMIOPort  Port=2  Side=Right
  connections:
  Rs1/LConn1 -- Conn1/RConn1
  LC Branch1/RConn1 -- Conn2/RConn1
  Rs1/RConn1 -- LC Branch1/LConn1

== system Coil5/stator winding model3/coil6 ==
  Ground : powerlib/Elements/Ground  DialogController=POWERSYS.PowerSysDialog  PhysicalDomain=powersysdomain  SubClassName=unknown  LeftPortType=p1  RightPortType=p1  LConnTagsString=a
  LC Branch1 : powerlib/Elements/Parallel RLC Branch  DialogController=POWERSYS.PowerSysDialog  PhysicalDomain=powersysdomain  SubClassName=unknown  LeftPortType=p1  RightPortType=p1  LConnTagsString=a  RConnTagsString=__new0  BranchType=RLC  Resistance=11.867e3/6  Inductance=(11.35E-3)/6  SetiL0=off  InitialCurrent=0  Capacitance=0.852e-9*6  Setx0=off  InitialVoltage=0  Measurements=None
  Rs1 : powerlib/Elements/Parallel RLC Branch  DialogController=POWERSYS.PowerSysDialog  PhysicalDomain=powersysdomain  SubClassName=unknown  LeftPortType=p1  RightPortType=p1  LConnTagsString=a  RConnTagsString=__new0  BranchType=R  Resistance=1.41/6  Inductance=1.0  SetiL0=off  InitialCurrent=0  Capacitance=1.0  Setx0=off  InitialVoltage=0  Measurements=None
  Conn1 : PMIOPort  Port=1  Side=Left
  Conn2 : PMIOPort  Port=2  Side=Right
  connections:
  Rs1/LConn1 -- Conn1/RConn1
  LC Branch1/RConn1 -- Conn2/RConn1
  Rs1/RConn1 -- LC Branch1/LConn1

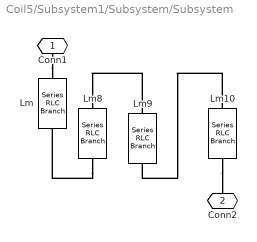
== system Coil5/Subsystem1/Subsystem/Subsystem ==
  Lm{,8..10} (4 alike) : powerlib/Elements/Series RLC Branch  DialogController=POWERSYS.PowerSysDialog  PhysicalDomain=powersysdomain  SubClassName=unknown  LeftPortType=p1  RightPortType=p1  LConnTagsString=__new0  RConnTagsString=__new0  BranchType=L  Resistance=1.0  Inductance=319e-3/(8*6*4)  SetiL0=off  InitialCurrent=0  Capacitance=1.0  Setx0=off  InitialVoltage=0  Measurements=None
  Conn1 : PMIOPort  Port=1  Side=Left
  Conn2 : PMIOPort  Port=2  Side=Right
  connections:
  Lm10/LConn1 -- Lm9/RConn1
  Lm9/LConn1 -- Lm8/LConn1
  Conn1/RConn1 -- Lm/LConn1
  Lm8/RConn1 -- Lm/RConn1
  Lm10/RConn1 -- Conn2/RConn1

== system Coil5/Subsystem2/Subsystem/Subsystem ==
  Lm{,8..10} (4 alike) : powerlib/Elements/Series RLC Branch  DialogController=POWERSYS.PowerSysDialog  PhysicalDomain=powersysdomain  SubClassName=unknown  LeftPortType=p1  RightPortType=p1  LConnTagsString=__new0  RConnTagsString=__new0  BranchType=L  Resistance=1.0  Inductance=319e-3/(8*6*4)  SetiL0=off  InitialCurrent=0  Capacitance=1.0  Setx0=off  InitialVoltage=0  Measurements=None
  Conn1 : PMIOPort  Port=1  Side=Left
  Conn2 : PMIOPort  Port=2  Side=Right
  connections:
  Lm10/LConn1 -- Lm9/RConn1
  Lm9/LConn1 -- Lm8/LConn1
  Conn1/RConn1 -- Lm/LConn1
  Lm8/RConn1 -- Lm/RConn1
  Lm10/RConn1 -- Conn2/RConn1

== system Coil5/Subsystem3/Subsystem/Subsystem ==
  Lm{,8..10} (4 alike) : powerlib/Elements/Series RLC Branch  DialogController=POWERSYS.PowerSysDialog  PhysicalDomain=powersysdomain  SubClassName=unknown  LeftPortType=p1  RightPortType=p1  LConnTagsString=__new0  RConnTagsString=__new0  BranchType=L  Resistance=1.0  Inductance=319e-3/(8*6*4)  SetiL0=off  InitialCurrent=0  Capacitance=1.0  Setx0=off  InitialVoltage=0  Measurements=None
  Conn1 : PMIOPort  Port=1  Side=Left
  Conn2 : PMIOPort  Port=2  Side=Right
  connections:
  Lm10/LConn1 -- Lm9/RConn1
  Lm9/LConn1 -- Lm8/LConn1
  Conn1/RConn1 -- Lm/LConn1
  Lm8/RConn1 -- Lm/RConn1
  Lm10/RConn1 -- Conn2/RConn1

== system Coil5/stator winding model2/coil5/Subsystem1 ==
  LC Branch1 : powerlib/Elements/Parallel RLC Branch  DialogController=POWERSYS.PowerSysDialog  PhysicalDomain=powersysdomain  SubClassName=unknown  LeftPortType=p1  RightPortType=p1  LConnTagsString=a  RConnTagsString=__new0  BranchType=RLC  Resistance=11.867e3/(6*8)  Inductance=(11.35E-3)/(6*8)  SetiL0=off  InitialCurrent=0  Capacitance=0.852e-9*(6*8)  Setx0=off  InitialVoltage=0  Measurements=None
  Rs1 : powerlib/Elements/Parallel RLC Branch  DialogController=POWERSYS.PowerSysDialog  PhysicalDomain=powersysdomain  SubClassName=unknown  LeftPortType=p1  RightPortType=p1  LConnTagsString=a  RConnTagsString=__new0  BranchType=R  Resistance=1.41/(6*8)  Inductance=1.0  SetiL0=off  InitialCurrent=0  Capacitance=1.0  Setx0=off  InitialVoltage=0  Measurements=None
  Conn2 : PMIOPort  Port=1  Side=Right
  Conn1 : PMIOPort  Port=2  Side=Left
  connections:
  Rs1/RConn1 -- LC Branch1/LConn1
  Rs1/LConn1 -- Conn1/RConn1
  LC Branch1/RConn1 -- Conn2/RConn1

== system Coil5/stator winding model2/coil5/Subsystem2 ==
  LC Branch1 : powerlib/Elements/Parallel RLC Branch  DialogController=POWERSYS.PowerSysDialog  PhysicalDomain=powersysdomain  SubClassName=unknown  LeftPortType=p1  RightPortType=p1  LConnTagsString=a  RConnTagsString=__new0  BranchType=RLC  Resistance=11.867e3/(6*8)  Inductance=(11.35E-3)/(6*8)  SetiL0=off  InitialCurrent=0  Capacitance=0.852e-9*(6*8)  Setx0=off  InitialVoltage=0  Measurements=None
  Rs1 : powerlib/Elements/Parallel RLC Branch  DialogController=POWERSYS.PowerSysDialog  PhysicalDomain=powersysdomain  SubClassName=unknown  LeftPortType=p1  RightPortType=p1  LConnTagsString=a  RConnTagsString=__new0  BranchType=R  Resistance=1.41/(6*8)  Inductance=1.0  SetiL0=off  InitialCurrent=0  Capacitance=1.0  Setx0=off  InitialVoltage=0  Measurements=None
  Conn2 : PMIOPort  Port=1  Side=Right
  Conn1 : PMIOPort  Port=2  Side=Left
  connections:
  Rs1/RConn1 -- LC Branch1/LConn1
  Rs1/LConn1 -- Conn1/RConn1
  LC Branch1/RConn1 -- Conn2/RConn1

== system Coil5/stator winding model2/coil5/Subsystem3 ==
  LC Branch1 : powerlib/Elements/Parallel RLC Branch  DialogController=POWERSYS.PowerSysDialog  PhysicalDomain=powersysdomain  SubClassName=unknown  LeftPortType=p1  RightPortType=p1  LConnTagsString=a  RConnTagsString=__new0  BranchType=RLC  Resistance=11.867e3/(6*8)  Inductance=(11.35E-3)/(6*8)  SetiL0=off  InitialCurrent=0  Capacitance=0.852e-9*(6*8)  Setx0=off  InitialVoltage=0  Measurements=None
  Rs1 : powerlib/Elements/Parallel RLC Branch  DialogController=POWERSYS.PowerSysDialog  PhysicalDomain=powersysdomain  SubClassName=unknown  LeftPortType=p1  RightPortType=p1  LConnTagsString=a  RConnTagsString=__new0  BranchType=R  Resistance=1.41/(6*8)  Inductance=1.0  SetiL0=off  InitialCurrent=0  Capacitance=1.0  Setx0=off  InitialVoltage=0  Measurements=None
  Conn2 : PMIOPort  Port=1  Side=Right
  Conn1 : PMIOPort  Port=2  Side=Left
  connections:
  Rs1/RConn1 -- LC Branch1/LConn1
  Rs1/LConn1 -- Conn1/RConn1
  LC Branch1/RConn1 -- Conn2/RConn1

== system Coil5/stator winding model2/coil5/Subsystem4 ==
  LC Branch1 : powerlib/Elements/Parallel RLC Branch  DialogController=POWERSYS.PowerSysDialog  PhysicalDomain=powersysdomain  SubClassName=unknown  LeftPortType=p1  RightPortType=p1  LConnTagsString=a  RConnTagsString=__new0  BranchType=RLC  Resistance=11.867e3/(6*8)  Inductance=(11.35E-3)/(6*8)  SetiL0=off  InitialCurrent=0  Capacitance=0.852e-9*(6*8)  Setx0=off  InitialVoltage=0  Measurements=None
  Rs1 : powerlib/Elements/Parallel RLC Branch  DialogController=POWERSYS.PowerSysDialog  PhysicalDomain=powersysdomain  SubClassName=unknown  LeftPortType=p1  RightPortType=p1  LConnTagsString=a  RConnTagsString=__new0  BranchType=R  Resistance=1.41/(6*8)  Inductance=1.0  SetiL0=off  InitialCurrent=0  Capacitance=1.0  Setx0=off  InitialVoltage=0  Measurements=None
  Conn2 : PMIOPort  Port=1  Side=Right
  Conn1 : PMIOPort  Port=2  Side=Left
  connections:
  Rs1/RConn1 -- LC Branch1/LConn1
  Rs1/LConn1 -- Conn1/RConn1
  LC Branch1/RConn1 -- Conn2/RConn1

== system Coil5/stator winding model2/coil5/Subsystem5 ==
  LC Branch1 : powerlib/Elements/Parallel RLC Branch  DialogController=POWERSYS.PowerSysDialog  PhysicalDomain=powersysdomain  SubClassName=unknown  LeftPortType=p1  RightPortType=p1  LConnTagsString=a  RConnTagsString=__new0  BranchType=RLC  Resistance=11.867e3/(6*8)  Inductance=(11.35E-3)/(6*8)  SetiL0=off  InitialCurrent=0  Capacitance=0.852e-9*(6*8)  Setx0=off  InitialVoltage=0  Measurements=None
  Rs1 : powerlib/Elements/Parallel RLC Branch  DialogController=POWERSYS.PowerSysDialog  PhysicalDomain=powersysdomain  SubClassName=unknown  LeftPortType=p1  RightPortType=p1  LConnTagsString=a  RConnTagsString=__new0  BranchType=R  Resistance=1.41/(6*8)  Inductance=1.0  SetiL0=off  InitialCurrent=0  Capacitance=1.0  Setx0=off  InitialVoltage=0  Measurements=None
  Conn2 : PMIOPort  Port=1  Side=Right
  Conn1 : PMIOPort  Port=2  Side=Left
  connections:
  Rs1/RConn1 -- LC Branch1/LConn1
  Rs1/LConn1 -- Conn1/RConn1
  LC Branch1/RConn1 -- Conn2/RConn1

== system Coil5/stator winding model2/coil5/Subsystem6 ==
  LC Branch1 : powerlib/Elements/Parallel RLC Branch  DialogController=POWERSYS.PowerSysDialog  PhysicalDomain=powersysdomain  SubClassName=unknown  LeftPortType=p1  RightPortType=p1  LConnTagsString=a  RConnTagsString=__new0  BranchType=RLC  Resistance=11.867e3/(6*8)  Inductance=(11.35E-3)/(6*8)  SetiL0=off  InitialCurrent=0  Capacitance=0.852e-9*(6*8)  Setx0=off  InitialVoltage=0  Measurements=None
  Rs1 : powerlib/Elements/Parallel RLC Branch  DialogController=POWERSYS.PowerSysDialog  PhysicalDomain=powersysdomain  SubClassName=unknown  LeftPortType=p1  RightPortType=p1  LConnTagsString=a  RConnTagsString=__new0  BranchType=R  Resistance=1.41/(6*8)  Inductance=1.0  SetiL0=off  InitialCurrent=0  Capacitance=1.0  Setx0=off  InitialVoltage=0  Measurements=None
  Conn2 : PMIOPort  Port=1  Side=Right
  Conn1 : PMIOPort  Port=2  Side=Left
  connections:
  Rs1/RConn1 -- LC Branch1/LConn1
  Rs1/LConn1 -- Conn1/RConn1
  LC Branch1/RConn1 -- Conn2/RConn1

== system Coil5/stator winding model2/coil5/Subsystem7 ==
  LC Branch1 : powerlib/Elements/Parallel RLC Branch  DialogController=POWERSYS.PowerSysDialog  PhysicalDomain=powersysdomain  SubClassName=unknown  LeftPortType=p1  RightPortType=p1  LConnTagsString=a  RConnTagsString=__new0  BranchType=RLC  Resistance=11.867e3/(6*8)  Inductance=(11.35E-3)/(6*8)  SetiL0=off  InitialCurrent=0  Capacitance=0.852e-9*(6*8)  Setx0=off  InitialVoltage=0  Measurements=None
  Rs1 : powerlib/Elements/Parallel RLC Branch  DialogController=POWERSYS.PowerSysDialog  PhysicalDomain=powersysdomain  SubClassName=unknown  LeftPortType=p1  RightPortType=p1  LConnTagsString=a  RConnTagsString=__new0  BranchType=R  Resistance=1.41/(6*8)  Inductance=1.0  SetiL0=off  InitialCurrent=0  Capacitance=1.0  Setx0=off  InitialVoltage=0  Measurements=None
  Conn2 : PMIOPort  Port=1  Side=Right
  Conn1 : PMIOPort  Port=2  Side=Left
  connections:
  Rs1/RConn1 -- LC Branch1/LConn1
  Rs1/LConn1 -- Conn1/RConn1
  LC Branch1/RConn1 -- Conn2/RConn1

== system Coil5/stator winding model2/coil5/Subsystem8 ==
  LC Branch1 : powerlib/Elements/Parallel RLC Branch  DialogController=POWERSYS.PowerSysDialog  PhysicalDomain=powersysdomain  SubClassName=unknown  LeftPortType=p1  RightPortType=p1  LConnTagsString=a  RConnTagsString=__new0  BranchType=RLC  Resistance=11.867e3/(6*8)  Inductance=(11.35E-3)/(6*8)  SetiL0=off  InitialCurrent=0  Capacitance=0.852e-9*(6*8)  Setx0=off  InitialVoltage=0  Measurements=None
  Rs1 : powerlib/Elements/Parallel RLC Branch  DialogController=POWERSYS.PowerSysDialog  PhysicalDomain=powersysdomain  SubClassName=unknown  LeftPortType=p1  RightPortType=p1  LConnTagsString=a  RConnTagsString=__new0  BranchType=R  Resistance=1.41/(6*8)  Inductance=1.0  SetiL0=off  InitialCurrent=0  Capacitance=1.0  Setx0=off  InitialVoltage=0  Measurements=None
  Conn2 : PMIOPort  Port=1  Side=Right
  Conn1 : PMIOPort  Port=2  Side=Left
  connections:
  Rs1/RConn1 -- LC Branch1/LConn1
  Rs1/LConn1 -- Conn1/RConn1
  LC Branch1/RConn1 -- Conn2/RConn1
